simulink model "testYarpSendDicts_cpp"  (R2016a)
settings: Solver=FixedStepDiscrete  StartTime=0.0  StopTime=inf  FixedStep=0.001  RelTol=1e-3
model workspace (MAT data in the model file):
  gtest = 0
undefined symbols (not defined in the file or in its folder): amplitude, pitch, valence, x, y, z
libraries: mnmBlocks x1
settings Model: Creator=Ulysses  LastModifiedBy=Ulysses
settings SolverCC: EnableConcurrentExecution=on
settings DataIOCC: LimitDataPoints=on  SaveFormat=StructureWithTime
settings OptimizationCC: BlockReduction=off  OptimizeBlockIOStorage=off  BufferReuse=off  GlobalBufferReuse=off  ExpressionFolding=off  LocalBlockOutputs=off
settings DebuggingCC: SolverPrmCheckMsg=warning  AllowSymbolicDim=off
settings HardwareCC: TargetBitPerLong=64  TargetBitPerPointer=64  TargetIntDivRoundTo=Zero  TargetEndianess=LittleEndian  TargetWordSize=64  TargetHWDeviceType=Intel->x86-64
settings ModelReferenceCC: PropagateSignalLabelsOutOfModel=off
settings RTWCC: Description=Generic Real-Time Target  BuildConfiguration=Faster Runs  TargetLang=C++
settings RTWCC: CustomInclude=|
  | C:\src\yarp-git_VS15_64bit\src\libYARP_OS\include
  | C:\src\yarp-git_VS15_64bit\src\libyarpc
  | C:\src\yarp-git_VS15_64bit\generated_include
settings RTWCC: CustomLibrary=|
  | C:\src\yarp-git_VS15_64bit\lib\Release\YARP_dev.lib
  | C:\src\yarp-git_VS15_64bit\lib\Release\YARP_init.lib
  | C:\src\yarp-git_VS15_64bit\lib\Release\YARP_OS.lib
  | C:\src\yarp-git_VS15_64bit\lib\Release\YARP_sig.lib
settings CodeAppCC: MaxIdLength=95
settings GRTTargetCC: GeneratePreprocessorConditionals=Use local settings  MatFileLogging=off  MultiInstanceERTCode=on  CodeInterfacePackaging=C++ class
settings ConfigComp: CovModelRefEnable=Off  CovSFcnEnable=off

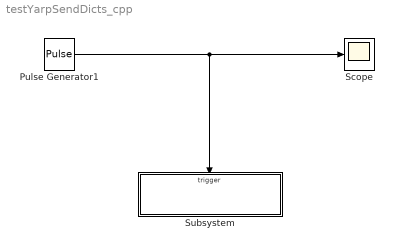
== system testYarpSendDicts_cpp ==
  Pulse Generator1 : DiscretePulseGenerator  PulseType=Time based  Period=10  PulseWidth=50
  Scope : Scope
  Subsystem : Subsystem
  wires:
  Pulse Generator1/1 -> Scope/1, Subsystem/Trigger

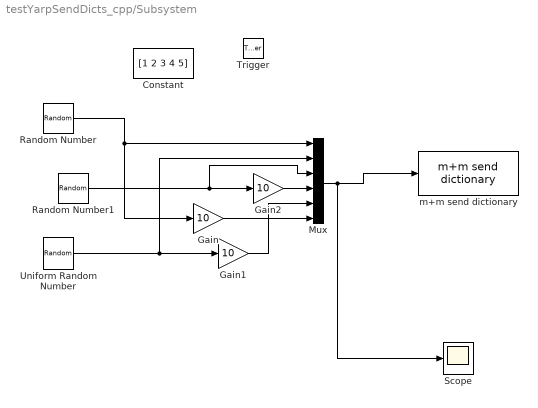
== system testYarpSendDicts_cpp/Subsystem ==
  Trigger : TriggerPort  VariantControl=Variant  PortDimensions=1
  Constant : Constant  Value=[1 2 3 4 5]
  Gain : Gain  Gain=10
  Gain1 : Gain  Gain=10
  Gain2 : Gain  Gain=10
  Mux : Mux  Inputs=6
  Random Number : RandomNumber  Mean=5
  Random Number1 : RandomNumber  Mean=5
  Scope : Scope
  Uniform Random Number : UniformRandomNumber  Minimum=-5
  m+m send dictionary : mnmBlocks/m+m send dictionary  msgFormat=x;y;z;amplitude;pitch;valence  portOut=/sim/sndstim/out  portIn=/sim/sndstim/in
  wires:
  Mux/1 -> Scope/1, m+m send dictionary/1
  Random Number/1 -> Gain/1, Mux/1
  Gain/1 -> Mux/6
  Uniform Random Number/1 -> Gain1/1, Mux/2
  Gain1/1 -> Mux/5
  Random Number1/1 -> Gain2/1, Mux/3
  Gain2/1 -> Mux/4
